simulink model "px4demo_fcn_call_uorb_example"  (R2017b)
settings: Solver=FixedStepDiscrete  StartTime=0.0  StopTime=inf  RelTol=1e-3  EnableMultiTasking=on
libraries: pixhawk_slib_uORB_RW x2, simulink x1
Description:
  | PX4 PSP Demo - Function Call uORB Example
  | 
  | This model demonstrates a function-call subsystem approach to modeling using triggered subsystems
  | 
  | This can be used to model this type of control architecture seen here:
  | https://github.com/PX4/Firmware/blob/master/src/modules/mc_att_control/mc_att_control_main.cpp
  | 
  | In the scheme described by the above source file, the control algorithm is driven by sensor updates. A variable is used to keep track of the time between updates such that the control terms such as Derivative and Integral can be computed accurately. Although these sensor updates are configured to come in at regular intervals, this approach accounts for any small differences in time due to jitter inprecision.
  | 
  | A similar approach can be modelled in Simulink. Inside the function-call subsystem, we read out the data from the sensor update event from a source block. The data can then be subsequently processed upon reception of the data. Because of this control structure, this event-driven control logic is considered to be asynchronous. If you check the sample times of the model you can see that this subsystem is configured this way
  | 
  | NOTE: This model is to be demosntrated in external mode. An alternative to being able to view these values without external mode is to modify this example to print the signals to the Nuttshell terminal using the print block
settings Model: SimulationMode=external  Creator=darenlee  LastModifiedBy=dream
settings SolverCC: PositivePriorityOrder=on
settings DataIOCC: LimitDataPoints=on  SaveFormat=StructureWithTime
settings OptimizationCC: DefaultParameterBehavior=Inlined  LifeSpan=1  MaxStackSize=64
settings DebuggingCC: AllowSymbolicDim=off  SFUnexpectedBacktrackingDiag=warning  SFNoUnconditionalDefaultTransitionDiag=warning  SFExecutionAtInitializationDiag=none
settings HardwareCC: ProdBitPerPointer=32  ProdBitPerSizeT=32  ProdBitPerPtrDiffT=32  ProdLargestAtomicInteger=Long  ProdLargestAtomicFloat=Double  ProdWordSize=32  ProdHWDeviceType=ARM Compatible->ARM Cortex
settings ModelReferenceCC: PropagateSignalLabelsOutOfModel=off
settings SFSimCC: MATLABDynamicMemAlloc=off
settings RTWCC: SystemTargetFile=ert.tlc  HardwareBoard=Pixhawk PX4  TemplateMakefile=ert_default_tmf  GenerateReport=on  Toolchain=Pixhawk Toolchain  IncludeHyperlinkInReport=on  LaunchReport=on  GenerateTraceInfo=on  GenerateTraceReport=on  GenerateTraceReportSl=on  GenerateTraceReportSf=on  GenerateTraceReportEml=on
settings CodeAppCC: IgnoreCustomStorageClasses=off  StateflowObjectComments=on
settings ERTTargetCC: MultiwordLength=2048  ExtMode=on  ExtModeTransport=1  ExtModeMexFile=ext_serial_win32_comm  ExtModeMexArgs=1 7 115200  ERTCustomFileTemplate=px4_codertarget_file_process.tlc  ConvertIfToSwitch=off  SuppressUnreachableDefaultCases=off
settings ConfigComp: CovMetricSettings=dw  CovHtmlReporting=on  CovSaveCumulativeToWorkspaceVar=on  CovSaveSingleToWorkspaceVar=on  CovExternalEMLEnable=off

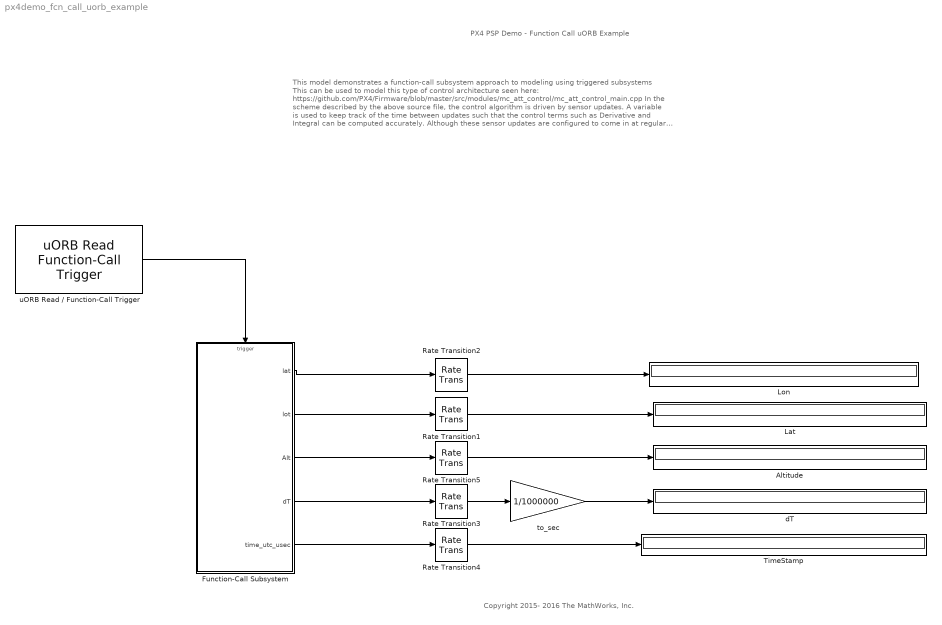
== system px4demo_fcn_call_uorb_example ==
  note: This model demonstrates a function-call subsystem approach to modeling using triggered subsystems
      |
      | This can be used to model this type of control architecture seen here:
      | https://github.com/PX4/Firmware/blob/master/src/modules/mc_att_control/mc_att_control_main.cpp
      |
      | In the scheme described by the above source file, the control algorithm is driven by sensor updates. A variable is used to keep track of the time between updates such that the control terms such as Derivative and Integral can be computed accurately. Although these sensor updates are configured to come in at regular intervals, this approach accounts for any small differences in time due to jitter inprecision.
      |
      | A similar approach can be modelled in Simulink. Inside the function-call subsystem, we read out the data from the sensor update event from a source block. The data can then be subsequently processed upon reception of the data. Because of this control structure, this event-driven control logic is considered to be asynchronous. If you check the sample times of the model you can see that this subsystem is configured this way
      |
      | NOTE: This model is to be demosntrated in external mode. An alternative to being able to view these values without external mode is to modify this example to print the signals to the Nuttshell terminal using the print block
  note: PX4 PSP Demo - Function Call uORB Example
  note: Copyright 2015- 2016 The MathWorks, Inc.
  Altitude : Display
  Function-Call Subsystem : Subsystem  TreatAsAtomicUnit=on
  Lat : Display
  Lon : Display
  Rate Transition{1..5} (5 alike) : RateTransition  Deterministic=off  OutPortSampleTime=0.1
  TimeStamp : Display
      settings: Format=long_e
  dT : Display
  to_sec : Gain  Gain=1/1000000  OutDataTypeStr=double
  uORB Read / Function-Call Trigger : pixhawk_slib_uORB_RW/uORB Read Function-Call Trigger  uORB_Topic_str='vehicle_gps_position'  BusObjVar=Bus: vehicle_gps_position_SL  uORB_Interval=1  AsyncOutput=on  Fcn_call_select=Generate Function Call Signal  TaskName='Task1'  Poll_timeout=100  Ts=-1
      settings: SourceProductName=Pixhawk Target Blocks
  wires:
  Function-Call Subsystem/1(lat) -> Rate Transition2/1
  Function-Call Subsystem/2(lot) -> Rate Transition1/1
  Function-Call Subsystem/3(Alt) -> Rate Transition5/1
  Rate Transition3/1 -> to_sec/1
  Rate Transition2/1 -> Lon/1
  Rate Transition1/1 -> Lat/1
  to_sec/1 -> dT/1
  uORB Read / Function-Call Trigger/1 -> Function-Call Subsystem/Trigger
  Rate Transition5/1 -> Altitude/1
  Function-Call Subsystem/4(dT) -> Rate Transition3/1
  Function-Call Subsystem/5(time_utc_usec) -> Rate Transition4/1
  Rate Transition4/1 -> TimeStamp/1

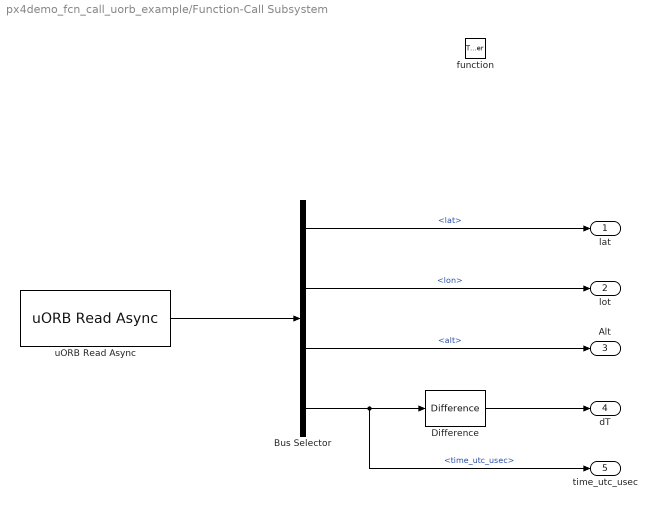
== system px4demo_fcn_call_uorb_example/Function-Call Subsystem ==
  function : TriggerPort  TriggerType=function-call  VariantControl=Variant
  Bus Selector : BusSelector  OutputSignals=lat,lon,alt,time_utc_usec
  Difference : simulink/Discrete/Difference  ICPrevInput=0.0  OutMin=[]  OutMax=[]  OutDataType=fixdt(1, 16)  OutScaling=2^-10  DoSatur=off
  uORB Read Async : pixhawk_slib_uORB_RW/uORB Read Async  uORB_Topic_str='vehicle_gps_position'  BusObjVar=Bus: vehicle_gps_position_SL
      settings: SourceProductName=Pixhawk Target Blocks
  lat : Outport
  lot : Outport  Port=2
  Alt : Outport  Port=3
  dT : Outport  Port=4
  time_utc_usec : Outport  Port=5
  wires:
  Bus Selector/4 -> time_utc_usec/1, Difference/1  "<time_utc_usec>"
  uORB Read Async/1 -> Bus Selector/1
  Bus Selector/1 -> lat/1  "<lat>"
  Bus Selector/2 -> lot/1  "<lon>"
  Bus Selector/3 -> Alt/1  "<alt>"
  Difference/1 -> dT/1
